simulink model "Exemplu_figura6"  (R2016a)
settings: Solver=VariableStepDiscrete  StartTime=0.0  StopTime=2080  RelTol=1e-3
undefined symbols (not defined in the file): m, n
settings Model: Creator=Cristina  LastModifiedBy=Cristina

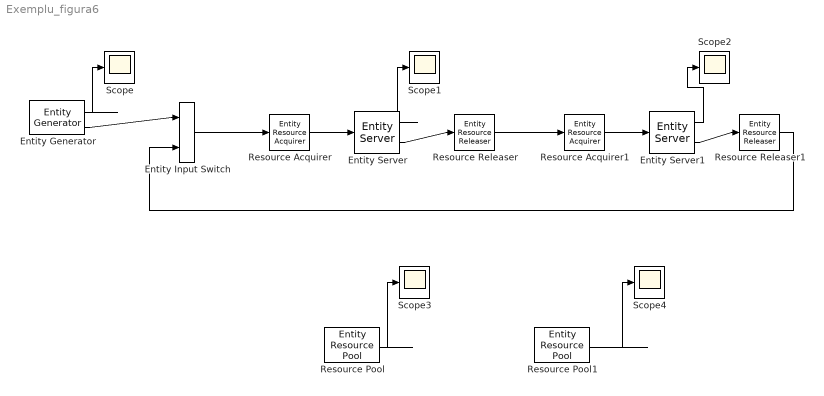
== system Exemplu_figura6 ==
  Entity Input Switch : EntityInputSwitch  InputPortMessageModes=m,m  OutputPortMessageModes=m
  Entity Generator : EntityGenerator  OutputPortMessageModes=n,m  TimeSource=MATLAB action  IntergenerationTimeAction=|  NumberEntitiesDeparted=on  EntityType=Structured  EntityTypeName=Entity
      | persistent count
      | if (isempty(count))
      |     count = 1;
      | end
      | if (count < 54)
      |     dt = 0;
      |     count = count + 1;
      | else
      |     dt = inf;
      | end
      settings: OutputPortMap=o0,o3
  Entity Server : EntityServer  InputPortMessageModes=m  OutputPortMessageModes=n,m  Capacity=50  ServiceTimeSource=MATLAB action  ServiceTimeAction=|  NumberEntitiesDeparted=on
      | persistent init
      | if (isempty(init))
      |     rng(379);
      |     init = true;
      | end
      | dt = 132 + 50 * rand;
      settings: OutputPortMap=o0,o9
  Entity Server1 : EntityServer  InputPortMessageModes=m  OutputPortMessageModes=n,m  Capacity=3  ServiceTimeSource=MATLAB action  ServiceTimeAction=|  NumberEntitiesDeparted=on
      | persistent init
      | if (isempty(init))
      |     rng(378);
      |     init = true;
      | end
      | dt = 4 + 6 * rand;
      settings: OutputPortMap=o0,o9
  Resource Acquirer : EntityResourceAcquirer  InputPortMessageModes=m  OutputPortMessageModes=m  NumberWaitingEntities=60  ResourceName=Machine
      settings: OutputPortMap=o3
  Resource Acquirer1 : EntityResourceAcquirer  InputPortMessageModes=m  OutputPortMessageModes=m  NumberWaitingEntities=60  ResourceName=Men
      settings: OutputPortMap=o3
  Resource Releaser : EntityResourceReleaser  InputPortMessageModes=m  OutputPortMessageModes=m  ResourceToRelease=Selected  ResourceName=Machine
  Resource Releaser1 : EntityResourceReleaser  InputPortMessageModes=m  OutputPortMessageModes=m  ResourceToRelease=Selected  ResourceName=Men
  Resource Pool : EntityResourcePool  ResourceName=Machine  ResourceAmount=50  AmountInUse=on
  Resource Pool1 : EntityResourcePool  ResourceName=Men  ResourceAmount=3  AmountInUse=on
  Scope{,1..4} (5 alike) : Scope
  wires:
  Entity Generator/2 -> Entity Input Switch/1
  Entity Input Switch/1 -> Resource Acquirer/1
  Resource Acquirer/1 -> Entity Server/1
  Entity Server/2 -> Resource Releaser/1
  Resource Releaser/1 -> Resource Acquirer1/1
  Resource Acquirer1/1 -> Entity Server1/1
  Entity Server1/2 -> Resource Releaser1/1
  Resource Releaser1/1 -> Entity Input Switch/2
  Entity Generator/1 -> Scope/1
  Entity Server/1 -> Scope1/1
  Entity Server1/1 -> Scope2/1
  Resource Pool/1 -> Scope3/1
  Resource Pool1/1 -> Scope4/1
